simulink model "MBD_UseCasesL"  (R2025a)
settings: Solver=VariableStepAuto  StartTime=0.0  StopTime=10.0  RelTol=1e-3
libraries: simulink x1
settings Model: Creator=mahij  LastModifiedBy=mahij

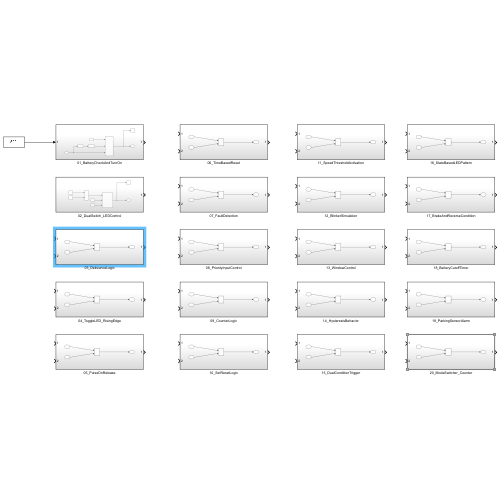
[thumbnail: Simulink's stored preview of the top-level diagram]
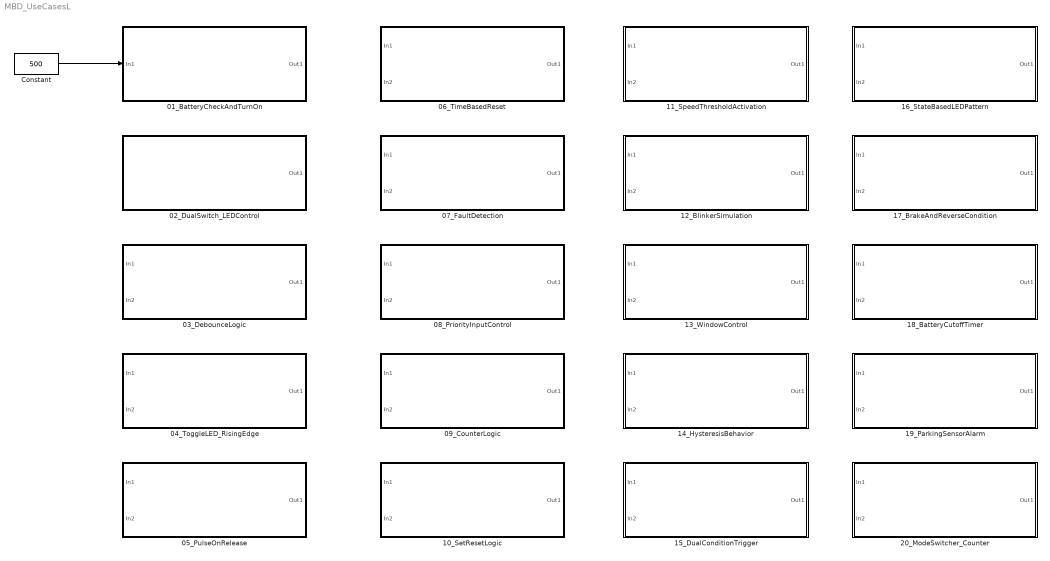
== system MBD_UseCasesL ==
  01_BatteryCheckAndTurnOn : Subsystem
  02_DualSwitch_LEDControl : Subsystem
  03_DebounceLogic : Subsystem
  04_ToggleLED_RisingEdge : Subsystem
  05_PulseOnRelease : Subsystem
  06_TimeBasedReset : Subsystem
  07_FaultDetection : Subsystem
  08_PriorityInputControl : Subsystem
  09_CounterLogic : Subsystem
  10_SetResetLogic : Subsystem
  11_SpeedThresholdActivation : Subsystem
  12_BlinkerSimulation : Subsystem
  13_WindowControl : Subsystem
  14_HysteresisBehavior : Subsystem
  15_DualConditionTrigger : Subsystem
  16_StateBasedLEDPattern : Subsystem
  17_BrakeAndReverseCondition : Subsystem
  18_BatteryCutoffTimer : Subsystem
  19_ParkingSensorAlarm : Subsystem
  20_ModeSwitcher_Counter : Subsystem
  Constant : Constant  Value=500
  wires:
  Constant/1 -> 01_BatteryCheckAndTurnOn/1(In1)

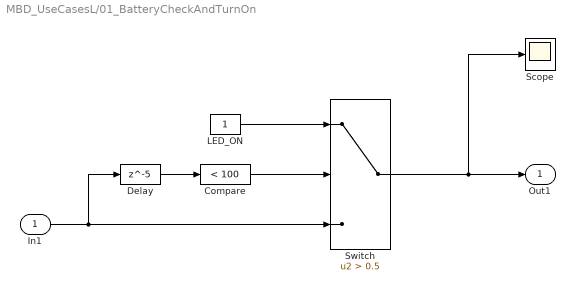
== system MBD_UseCasesL/01_BatteryCheckAndTurnOn ==
  In1 : Inport
  Compare : simulink/Logic and Bit Operations/Compare To Constant  relop=<  const=100  OutDataTypeStr=boolean
  Delay : Delay  DelayLength=5
  LED_ON : Constant
  Scope : Scope
      settings: ActiveDisplayYMinimum=-949.08651690821239  ActiveDisplayYMaximum=689.313483091787
  Switch : Switch  Criteria=u2 > Threshold  Threshold=0.5  SaturateOnIntegerOverflow=off  InputSameDT=off
  Out1 : Outport
  wires:
  In1/1 -> Delay/1, Switch/3
  Delay/1 -> Compare/1
  Compare/1 -> Switch/2
  LED_ON/1 -> Switch/1
  Switch/1 -> Scope/1, Out1/1

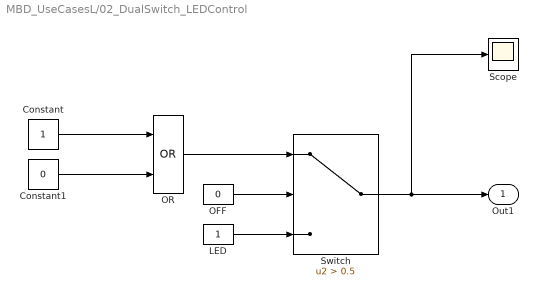
== system MBD_UseCasesL/02_DualSwitch_LEDControl ==
  Constant : Constant
  Constant1 : Constant  Value=0
  LED : Constant
  OFF : Constant  Value=0
  OR : Logic  Operator=OR  AllPortsSameDT=off  OutDataTypeStr=boolean
  Scope : Scope
      settings: ActiveDisplayYMinimum=0.9  ActiveDisplayYMaximum=1.1
  Switch : Switch  Criteria=u2 > Threshold  Threshold=0.5  SaturateOnIntegerOverflow=off  InputSameDT=off
  Out1 : Outport
  wires:
  Constant/1 -> OR/1
  Constant1/1 -> OR/2
  OR/1 -> Switch/1
  OFF/1 -> Switch/2
  LED/1 -> Switch/3
  Switch/1 -> Scope/1, Out1/1

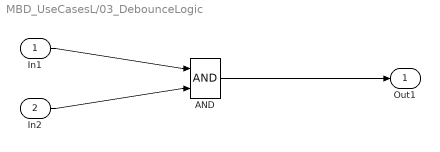
== system MBD_UseCasesL/03_DebounceLogic ==
  In1 : Inport
  In2 : Inport  Port=2
  AND : Logic  AllPortsSameDT=off  OutDataTypeStr=boolean
  Out1 : Outport
  wires:
  In1/1 -> AND/1
  In2/1 -> AND/2
  AND/1 -> Out1/1

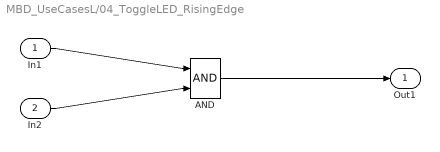
== system MBD_UseCasesL/04_ToggleLED_RisingEdge ==
  In1 : Inport
  In2 : Inport  Port=2
  AND : Logic  AllPortsSameDT=off  OutDataTypeStr=boolean
  Out1 : Outport
  wires:
  In1/1 -> AND/1
  In2/1 -> AND/2
  AND/1 -> Out1/1

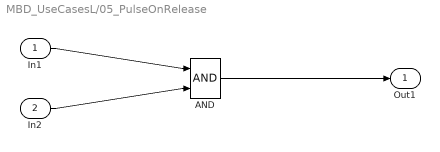
== system MBD_UseCasesL/05_PulseOnRelease ==
  In1 : Inport
  In2 : Inport  Port=2
  AND : Logic  AllPortsSameDT=off  OutDataTypeStr=boolean
  Out1 : Outport
  wires:
  In1/1 -> AND/1
  In2/1 -> AND/2
  AND/1 -> Out1/1

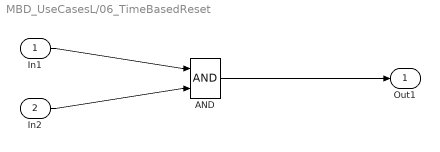
== system MBD_UseCasesL/06_TimeBasedReset ==
  In1 : Inport
  In2 : Inport  Port=2
  AND : Logic  AllPortsSameDT=off  OutDataTypeStr=boolean
  Out1 : Outport
  wires:
  In1/1 -> AND/1
  In2/1 -> AND/2
  AND/1 -> Out1/1

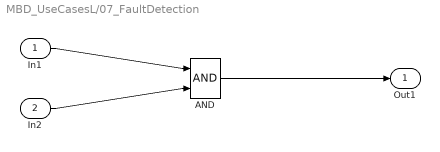
== system MBD_UseCasesL/07_FaultDetection ==
  In1 : Inport
  In2 : Inport  Port=2
  AND : Logic  AllPortsSameDT=off  OutDataTypeStr=boolean
  Out1 : Outport
  wires:
  In1/1 -> AND/1
  In2/1 -> AND/2
  AND/1 -> Out1/1

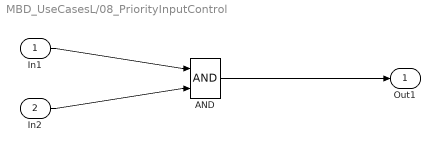
== system MBD_UseCasesL/08_PriorityInputControl ==
  In1 : Inport
  In2 : Inport  Port=2
  AND : Logic  AllPortsSameDT=off  OutDataTypeStr=boolean
  Out1 : Outport
  wires:
  In1/1 -> AND/1
  In2/1 -> AND/2
  AND/1 -> Out1/1

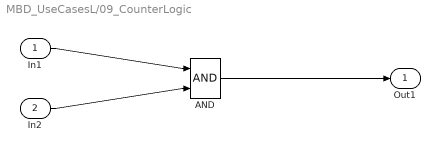
== system MBD_UseCasesL/09_CounterLogic ==
  In1 : Inport
  In2 : Inport  Port=2
  AND : Logic  AllPortsSameDT=off  OutDataTypeStr=boolean
  Out1 : Outport
  wires:
  In1/1 -> AND/1
  In2/1 -> AND/2
  AND/1 -> Out1/1

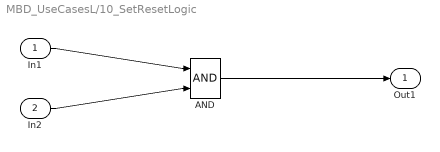
== system MBD_UseCasesL/10_SetResetLogic ==
  In1 : Inport
  In2 : Inport  Port=2
  AND : Logic  AllPortsSameDT=off  OutDataTypeStr=boolean
  Out1 : Outport
  wires:
  In1/1 -> AND/1
  In2/1 -> AND/2
  AND/1 -> Out1/1

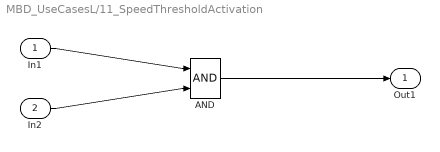
== system MBD_UseCasesL/11_SpeedThresholdActivation ==
  In1 : Inport
  In2 : Inport  Port=2
  AND : Logic  AllPortsSameDT=off  OutDataTypeStr=boolean
  Out1 : Outport
  wires:
  In1/1 -> AND/1
  In2/1 -> AND/2
  AND/1 -> Out1/1

== system MBD_UseCasesL/12_BlinkerSimulation ==
  In1 : Inport
  In2 : Inport  Port=2
  AND : Logic  AllPortsSameDT=off  OutDataTypeStr=boolean
  Out1 : Outport
  wires:
  In1/1 -> AND/1
  In2/1 -> AND/2
  AND/1 -> Out1/1

== system MBD_UseCasesL/13_WindowControl ==
  In1 : Inport
  In2 : Inport  Port=2
  AND : Logic  AllPortsSameDT=off  OutDataTypeStr=boolean
  Out1 : Outport
  wires:
  In1/1 -> AND/1
  In2/1 -> AND/2
  AND/1 -> Out1/1

== system MBD_UseCasesL/14_HysteresisBehavior ==
  In1 : Inport
  In2 : Inport  Port=2
  AND : Logic  AllPortsSameDT=off  OutDataTypeStr=boolean
  Out1 : Outport
  wires:
  In1/1 -> AND/1
  In2/1 -> AND/2
  AND/1 -> Out1/1

== system MBD_UseCasesL/15_DualConditionTrigger ==
  In1 : Inport
  In2 : Inport  Port=2
  AND : Logic  AllPortsSameDT=off  OutDataTypeStr=boolean
  Out1 : Outport
  wires:
  In1/1 -> AND/1
  In2/1 -> AND/2
  AND/1 -> Out1/1

== system MBD_UseCasesL/16_StateBasedLEDPattern ==
  In1 : Inport
  In2 : Inport  Port=2
  AND : Logic  AllPortsSameDT=off  OutDataTypeStr=boolean
  Out1 : Outport
  wires:
  In1/1 -> AND/1
  In2/1 -> AND/2
  AND/1 -> Out1/1

== system MBD_UseCasesL/17_BrakeAndReverseCondition ==
  In1 : Inport
  In2 : Inport  Port=2
  AND : Logic  AllPortsSameDT=off  OutDataTypeStr=boolean
  Out1 : Outport
  wires:
  In1/1 -> AND/1
  In2/1 -> AND/2
  AND/1 -> Out1/1

== system MBD_UseCasesL/18_BatteryCutoffTimer ==
  In1 : Inport
  In2 : Inport  Port=2
  AND : Logic  AllPortsSameDT=off  OutDataTypeStr=boolean
  Out1 : Outport
  wires:
  In1/1 -> AND/1
  In2/1 -> AND/2
  AND/1 -> Out1/1

== system MBD_UseCasesL/19_ParkingSensorAlarm ==
  In1 : Inport
  In2 : Inport  Port=2
  AND : Logic  AllPortsSameDT=off  OutDataTypeStr=boolean
  Out1 : Outport
  wires:
  In1/1 -> AND/1
  In2/1 -> AND/2
  AND/1 -> Out1/1

== system MBD_UseCasesL/20_ModeSwitcher_Counter ==
  In1 : Inport
  In2 : Inport  Port=2
  AND : Logic  AllPortsSameDT=off  OutDataTypeStr=boolean
  Out1 : Outport
  wires:
  In1/1 -> AND/1
  In2/1 -> AND/2
  AND/1 -> Out1/1
